simulink model "Solar_model_try_5V"  (R2019a)
settings: Solver=VariableStepAuto  StartTime=0.0  StopTime=10.0  RelTol=1e-2
libraries: powerlib x10, simulink x2, re_lib x1, powerlib_meascontrol x1
settings Model: Creator=stushar  LastModifiedBy=stushar
settings SolverCC: AlgebraicLoopSolver=LineSearch

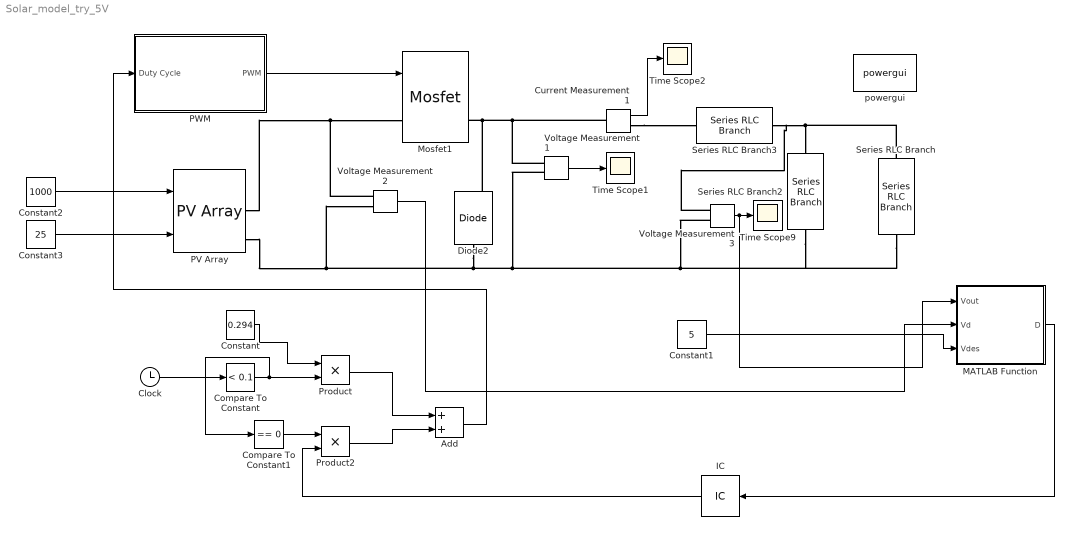
== system Solar_model_try_5V ==
  Add : Sum
  Clock : Clock
  Compare To Constant : simulink/Logic and Bit Operations/Compare To Constant  relop=<  const=0.1  OutDataTypeStr=boolean
  Compare To Constant1 : simulink/Logic and Bit Operations/Compare To Constant  relop===  const=0  OutDataTypeStr=boolean
  Constant : Constant  Value=0.294
  Constant1 : Constant  Value=5
  Constant2 : Constant  Value=1000
  Constant3 : Constant  Value=25
  Current Measurement1 : powerlib/Measurements/Current Measurement  PhasorSimulation=off  OutputType=Complex  PSBequivalent=0
      settings: SourceProductName=Simscape Electrical
  Diode2 : powerlib/Power Electronics/Diode  Ron=0.00001  Lon=0  Vf=0  IC=0  UseSnubber=off  Rs=500  Cs=250e-9  Measurements=on
      settings: SourceProductName=Simscape Electrical
  IC : InitialCondition
  MATLAB Function : MATLAB Function  TreatAsAtomicUnit=on
  Mosfet1 : powerlib/Power Electronics/Mosfet  Ron=0.0001  Lon=0  Rd=0.001  Vfd=0  IC=0  Rs=42  Cs=600e-12  Measurements=on
      settings: SourceProductName=Simscape Electrical
  PV Array : re_lib/Solar/PV Array  Npar=1  Nser=1  PlotType=array @ 1000 W/m2 & specified temperatures  S_vec="[ 1000  500  100 ]"  Temp_C_vec="[ 45 25  ]"  ModuleName=User-defined  PlotWhenSelected=off  Pm=87.348  Ncell=72  Voc=21.7  Isc=5.34  Vm=17.4  Im=5.02  beta_Voc_pc=-0.3783  alpha_Isc_pc=0.0397  beta_Voc=-0.082091  alpha_Isc=0.00212  IL=5.3513  I0=3.2286e-10  nI=0.49872  Rsh=434.5483  Rs=0.32346  BAL=off  Tc=1e-6  Tfilter=5e-5
      settings: SourceProductName=Simscape Electrical
  PWM : Subsystem
  Product : Product
  Product2 : Product
  Series RLC Branch : powerlib/Elements/Series RLC Branch  LConnTagsString=__new0  RConnTagsString=__new0  BranchType=R  Resistance=2.525  Inductance=1e-3  SetiL0=off  InitialCurrent=0  Capacitance=1e-6  Setx0=off  InitialVoltage=0  Measurements=None
      settings: SourceProductName=Simscape Electrical
  Series RLC Branch2 : powerlib/Elements/Series RLC Branch  LConnTagsString=__new0  RConnTagsString=__new0  BranchType=RC  Resistance=.003  Inductance=1e-3  SetiL0=off  InitialCurrent=0  Capacitance=100e-6  Setx0=on  InitialVoltage=0  Measurements=Branch voltage
      settings: SourceProductName=Simscape Electrical
  Series RLC Branch3 : powerlib/Elements/Series RLC Branch  LConnTagsString=__new0  RConnTagsString=__new0  BranchType=RL  Resistance=2.1e-3  Inductance=1000e-6  SetiL0=off  InitialCurrent=0  Capacitance=1e-6  Setx0=off  InitialVoltage=0  Measurements=None
      settings: SourceProductName=Simscape Electrical
  Time Scope1 : Scope
  Time Scope2 : Scope
  Time Scope9 : Scope
  Voltage Measurement1 : powerlib/Measurements/Voltage Measurement  PhasorSimulation=off  OutputType=Complex  PSBequivalent=0
      settings: SourceProductName=Simscape Electrical
  Voltage Measurement2 : powerlib/Measurements/Voltage Measurement  PhasorSimulation=off  OutputType=Complex  PSBequivalent=0
      settings: SourceProductName=Simscape Electrical
  Voltage Measurement3 : powerlib/Measurements/Voltage Measurement  PhasorSimulation=off  OutputType=Complex  PSBequivalent=0
      settings: SourceProductName=Simscape Electrical
  powergui : powerlib/powergui  Priority=1  SimulationMode=Discrete  SampleTime=10e-8  frequency=60  Iterations=50  frequencyindice=0  Pbase=100e6  ErrMax=1e-4  UnitsV=kV  UnitsW=MW  buscounter=0  FunctionMessages=off  echomessages=off  EnableUseOfTLC=off  CurrentSourceSwitches=off  DisableSnubberDevices=off  DisableRonSwitches=off  DisableVfSwitches=off  DisplayEquations=off  AutomaticDiscreteSolvers=off  SolverType=Tustin/Backward Euler (TBE)  Interpol=off  ExternalGateDelay=off  methode=off  Ts=100  x0status=blocks  SPID=off  SwTol=0  HookPort=off  NonlinearTolerance=0  nMaxIteration=15  ContinueOnMaxIteration=off  RestoreLinks=warning  ResistiveCurrentMeasurement=off  Frange=[0:2:500]  Ylog=off  Xlog=on  ShowGrid=off  save=off  variable=ZData  structure=0  ZoomFFT=off  StartTime=0.0  cycles=1  DisplayStyle=1  fundamental=60  FreqAxis=off  MaxFrequency=1000  frequencyindicesteady=1  RmsSteady=1  display=off
      settings: SourceProductName=Simscape Electrical
  wires:
  PWM/1(PWM) -> Mosfet1/1
  Compare To Constant/1 -> Compare To Constant1/1, Product/2
  IC/1 -> Product2/2
  Add/1 -> PWM/1("Duty Cycle ")
  Voltage Measurement1/1 -> Time Scope1/1
  Product2/1 -> Add/2
  Voltage Measurement2/1 -> MATLAB Function/2(Vd)
  Voltage Measurement3/1 -> MATLAB Function/1(Vout), Time Scope9/1
  Current Measurement1/1 -> Time Scope2/1
  Constant/1 -> Product/1
  Compare To Constant1/1 -> Product2/1
  Product/1 -> Add/1
  Clock/1 -> Compare To Constant/1
  Constant3/1 -> PV Array/2
  Constant2/1 -> PV Array/1
  MATLAB Function/1(D) -> IC/1
  Constant1/1 -> MATLAB Function/3(Vdes)
  connections:
  Voltage Measurement3/LConn2 -- Series RLC Branch/RConn1 -- Series RLC Branch2/RConn1 -- Voltage Measurement1/LConn2 -- Voltage Measurement2/LConn2 -- PV Array/RConn2 -- Diode2/LConn1
  Voltage Measurement1/LConn1 -- Current Measurement1/LConn1 -- Diode2/RConn1 -- Mosfet1/RConn1
  Voltage Measurement2/LConn1 -- PV Array/RConn1 -- Mosfet1/LConn1
  Series RLC Branch/LConn1 -- Series RLC Branch2/LConn1 -- Voltage Measurement3/LConn1 -- Series RLC Branch3/RConn1
  Current Measurement1/RConn1 -- Series RLC Branch3/LConn1

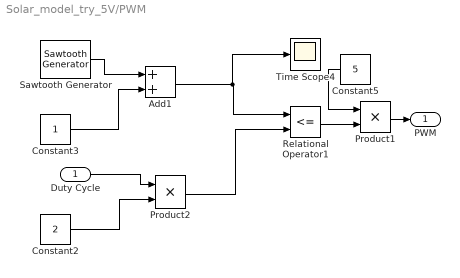
== system Solar_model_try_5V/PWM ==
  "Duty Cycle " : Inport
  Add1 : Sum
  Constant2 : Constant  Value=2
  Constant3 : Constant
  Constant5 : Constant  Value=5
  Product1 : Product
  Product2 : Product
  Relational Operator1 : RelationalOperator  Operator=<=  OutDataTypeStr=boolean  RndMeth=Nearest
  Sawtooth Generator : powerlib_meascontrol/Pulse & Signal Generators/Sawtooth Generator  Freq=40000  Phase=0  Ts=0
      settings: SourceProductName=Simscape Electrical
  Time Scope4 : Scope
  PWM : Outport
  wires:
  Relational Operator1/1 -> Product1/2
  Product2/1 -> Relational Operator1/2
  Sawtooth Generator/1 -> Add1/1
  Constant5/1 -> Product1/1
  Constant3/1 -> Add1/2
  Add1/1 -> Time Scope4/1, Relational Operator1/1
  Product1/1 -> PWM/1
  "Duty Cycle "/1 -> Product2/1
  Constant2/1 -> Product2/2

== matlab function Solar_model_try_5V/MATLAB Function ==
  data: D output; Vout input; Vd input; Vdes input
function D= fcn(Vout,Vd,Vdes)
SSE=0.312;
Vdes=Vdes+SSE;
Dgiven=Vdes/Vd;
Dfound=Vout/Vd;
%#codegen
Derror=(Dgiven-Dfound)/Dgiven;
SSE=Vdes-Vout;
VDES=Vdes-SSE;
SE=Vdes-Vout;
D=Dgiven/(1-Derror);
% if abs((Din*Vd)-SE))>abs((Din*Vd)+SE))
%     D=Din+E/Vd;
% else
%     D=Din-E/Vd;
% end
